simulink model "Part_C_Simulink"  (R2018b)
settings: Solver=VariableStepAuto  StartTime=0.0  StopTime=t_dur  MaxStep=t_step  RelTol=1e-3
values from neighbouring files (symbols this model uses):
  B = 21e-3    (= 0.021)    [Part_c.m]    (also in Part_d.m)
  freq = 112    [Part_c.m]    (also in Part_d.m)
  i_a = 1.7e3    (= 1700)    [Part_c.m]    (also in Part_d.m)
  l = 0.5    [Part_c.m]    (also in Part_d.m; Part_e_ramp.m; Part_e_step.m)
  N = 126    [Part_c.m]    (also in Part_d.m; Part_e_ramp.m; Part_e_step.m)
  r = 1/6    (= 0.166666666667)    [Part_c.m]    (also in Part_d.m; Part_e_ramp.m; Part_e_step.m)
libraries: simulink x1
settings Model: Creator=Nick Carcione  LastModifiedBy=Nick Carcione

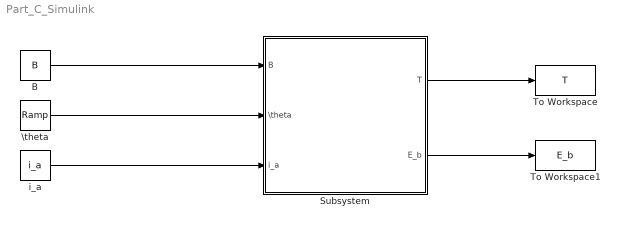
== system Part_C_Simulink ==
  B : Constant  Value=B
  Subsystem : Subsystem
  To Workspace : ToWorkspace  VariableName=T  SaveFormat=Timeseries  SampleTime=-1
  To Workspace1 : ToWorkspace  VariableName=E_b  SaveFormat=Timeseries  SampleTime=-1
  \theta : simulink/Sources/Ramp  slope=freq  start=0  InitialOutput=0
  i_a : Constant  Value=i_a
  wires:
  B/1 -> Subsystem/1(B)
  \theta/1 -> Subsystem/2(\theta)
  i_a/1 -> Subsystem/3(i_a)
  Subsystem/2(E_b) -> To Workspace1/1
  Subsystem/1(T) -> To Workspace/1

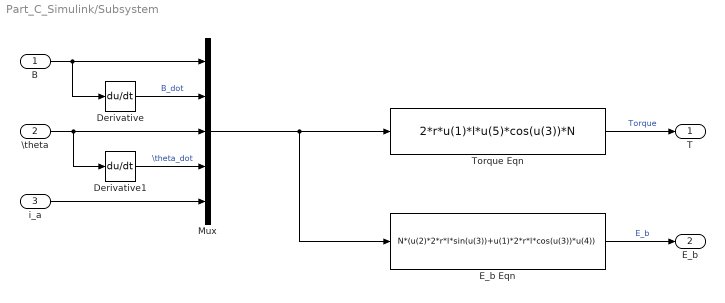
== system Part_C_Simulink/Subsystem ==
  B : Inport
  \theta : Inport  Port=2
  i_a : Inport  Port=3
  Derivative : Derivative
  Derivative1 : Derivative
  E_b Eqn : Fcn  Expr=N*(u(2)*2*r*l*sin(u(3))+u(1)*2*r*l*cos(u(3))*u(4))
  Mux : Mux  Inputs=5
  Torque Eqn : Fcn  Expr=2*r*u(1)*l*u(5)*cos(u(3))*N
  T : Outport
  E_b : Outport  Port=2
  wires:
  Mux/1 -> E_b Eqn/1, Torque Eqn/1
  B/1 -> Mux/1, Derivative/1
  \theta/1 -> Mux/3, Derivative1/1
  i_a/1 -> Mux/5
  Derivative1/1 -> Mux/4  "\\theta_dot"
  Derivative/1 -> Mux/2  "B_dot"
  Torque Eqn/1 -> T/1  "Torque"
  E_b Eqn/1 -> E_b/1  "E_b"
